simulink model "IEEE39bus"  (Simulink 8.5)
settings: Solver=ode3  SolverMode=SingleTasking  StartTime=0.0  StopTime=50  FixedStep=Ts  RelTol=1e-3
PostLoadFcn:
  | Ts=25e-6; IEEE39BusLineLength;
  | vNomHV = 345E3;fNom=50;load('Dynamicload.mat');
InitFcn:
  | Ts=25e-6; IEEE39BusLineLength;
  | vNomHV = 345E3;fNom=50;load('Dynamicload.mat');
undefined symbols (not defined in the file): D1, Delta, load15, load16, load18, load20, load21, load23, load24, load25, load26, load27, load28, load29, load3, load39, load4, load7, load8, TL_10_11_len, TL_10_13_len, TL_13_14_len, TL_14_15_len, TL_15_16_len, TL_16_17_len, TL_16_19_len, TL_16_21_len, TL_16_24_len, TL_17_18_len, TL_17_27_len, TL_1_2_len, TL_1_39_len, TL_21_22_len, TL_22_23_len, TL_24_23_len, TL_25_26_len, TL_26_27_len, TL_26_28_len, TL_26_29_len, TL_28_29_len, TL_2_25_len, TL_2_2_len, TL_3_18_len, TL_3_4_len, TL_4_14_len, TL_4_5_len, TL_5_6_len, TL_5_8_len, TL_6_11_len, TL_6_7_len, TL_7_8_len, TL_8_9_len, TL_9_39_len
libraries: powerlib x175, op_dpl_lib x34, rtlab x14, sps_avr x9, powerlib_extras x2, artemis x1, powerlib_meascontrol x1
(part 3 of 5)

== system IEEE39bus/SS_EastSystem1/GT 5 ==
  5 MW : powerlib/Elements/Three-Phase Parallel RLC Load  LConnTagsString=A|B|C  Configuration=Y (grounded)  NominalVoltage=22e3  NominalFrequency=50  ActivePower=5e6  InductivePower=0  CapacitivePower=0  Measurements=None  LoadType=constant Z
  Bus Selector1 : BusSelector  OutputSignals="dq0 components.Stator voltage  vq (pu),dq0 components.Stator voltage  vd (pu),Mechanical.Rotor speed  wm  (pu),Mechanical.Rotor speed deviation  dw (pu),Output active power   Peo (pu),Output reactive power  Qeo (pu)"
  Bus 34 : powerlib/Measurements/Three-Phase V-I Measurement  VoltageMeasurement=phase-to-ground  SetLabelV=on  LabelV=V_bus_G5  Vpu=off  VpuLL=off  CurrentMeasurement=no  SetLabelI=on  LabelI=I_bus_G5  Ipu=off  Pbase=100e6  Vbase=16.5e3  OutputType=Complex  PhasorSimulation=off  PSBequivalent=0
  Excitation System1 : sps_avr/Excitation System  tr=20e-3  reg=[ 200, 0.02 ]  exc=[ 1, 0 .19]  tgr=[ 0, 0 ]  damp=[ 0.0012, 1 ]  sat=[ 0, 0 ]  lim=[ 0, 7.32, 0 ]  v0=[1.0123 3.3412]
  GT1_CB6 : Subsystem
  Ground : Ground
  HTG : powerlib/Machines/Hydraulic Turbine and Governor  sm="[ 10/3  0.07 ]"  gate="[  0.01  0.97518  -0.1  0.1 ]"  reg="[  0.05  1.163  0.105  0  0.01  ]"  hyd="[  0  2.67  ]"  dref=0  po=0.709
  Load Flow Bus : powerlib/Measurements/Load Flow Bus  LConnTagsString=a  ID=Bus-34  Vbase=22000  Vref=1.0123  Vangle=0  VLF=1.012  angleLF=-37.01
      settings: AttributesFormatString=%<ID>\n%<Vbase>V\n%<VLF>pu\n%<angleLF>deg.
  Machine 5 520 MVA 22 kV : powerlib/Machines/Synchronous Machine pu Standard  PresetModel=No  MechanicalLoad=Mechanical power Pm  ShowDetailedParameters=on  RotorType=Round  Units=per unit standard parameters  MeasurementBus=off  NominalParameters="[ 520E6  22000   50 ]"  Reactances1=[ 3.484 0.686 0.343 3.224 0.8632 0.343 0.054 ]  Reactances2=[ 0.995, 0.195, 0.155, 0.568, 0.143, 0.16 ]  dAxisTimeConstants=Open-circuit  qAxisTimeConstants=Open-circuit  TimeConstants1=[]  TimeConstants2=[5.4 0.03 0.44 0.04]  TimeConstants3=[]  TimeConstants4=[]  TimeConstants5=[ 9.2, 0.01, 0.01 ]  TimeConstants6=[]  TimeConstants7=[]  TimeConstants8=[]  StatorResistance=0  Mechanical=[ 5 0.02 20]  PolePairs=20  InitialConditions=[0 -74.2196 0.822255 0.822255 0.822255 -56.5136 -176.514 63.4864 3.34118]  SetSaturation=off  Saturation=[0.6404,0.7127,0.8441,0.9214,0.9956,1.082,1.19,1.316,1.457;0.7,0.7698,0.8872,0.9466,0.9969,1.046,1.1,1.151,1.201]  LoadFlowParameters=[1 508000000 22270.6 0]  TsPowergui=0  TsBlock=-1  IterativeModel=Trapezoidal non iterative  BusType=PV  Pref=4.08e+008  Qref=0  Qmin=-300e6  Qmax=200e6  PLF=0  QLF=0
      settings: AttributesFormatString=\n\n
  Pref : Constant  Value=0.709
  Terminator5 : Terminator
  Transformer 5 572 MVA 22 kV / 345 kV : powerlib/Elements/Three-Phase Transformer (Two Windings)  Winding1Connection=Delta (D1)  Winding2Connection=Yg  CoreType=Three single-phase transformers  SetSaturation=off  Hysteresis=off  DataFile='hysteresis'  SetInitialFlux=off  Measurements=None  UNITS=pu  NominalPower=[ 572e6 50 ]  Winding1="[ 22e3 0.009*572/100/2    0.018*572/100/2]"  Winding2="[ 1.009*345e3 0.009*572/100/2    0.018*572/100/2]"  Rm=500  Lm=500  L0=0.5  Saturation="[ 0,0  ;  0.005,1.2  ;  1.0,1.4 ]"  InitialFluxes=[ 0.8 , -0.8 , 0.7 ]  MoreParameters=off  BreakLoop=off  DataType=off  TransfoNumber=0
  Vref : Constant  Value=1.0123
  wref : Constant
  A : PMIOPort  Port=1  Side=Right
  B : PMIOPort  Port=2  Side=Right
  C : PMIOPort  Port=3  Side=Right
  tag scope: P_G5=global, Q_G5=global, V_G5=global, Wm_G5=global
  wires:
  Ground/1 -> Excitation System1/4
  HTG/2 -> Terminator5/1
  Vref/1 -> Excitation System1/1
  Pref/1 -> HTG/2
  wref/1 -> HTG/1
  HTG/1 -> Machine 5 520 MVA 22 kV/1
  Machine 5 520 MVA 22 kV/1 -> Bus Selector1/1
  Bus Selector1/1 -> Excitation System1/3  "<Stator voltage  vq (pu)>"
  Bus Selector1/2 -> Excitation System1/2  "<Stator voltage  vd (pu)>"
  Bus Selector1/3 -> HTG/3, [Wm_G5]  "<Rotor speed  wm  (pu)>"
  Bus Selector1/4 -> HTG/5  "<Rotor speed deviation  dw (pu)>"
  Bus Selector1/5 -> HTG/4, [P_G5]  "<Output active power   Peo (pu)>"
  Bus Selector1/6 -> [Q_G5]  "<Output reactive power  Qeo (pu)>"
  [V_bus_G5] -> [V_G5]
  Excitation System1/1 -> Machine 5 520 MVA 22 kV/2
  connections:
  Transformer 5 572 MVA 22 kV / 345 kV/LConn1 -- Load Flow Bus/LConn1 -- Bus 34/RConn1 -- 5 MW/LConn1
  Transformer 5 572 MVA 22 kV / 345 kV/LConn2 -- Bus 34/RConn2 -- 5 MW/LConn2
  Transformer 5 572 MVA 22 kV / 345 kV/LConn3 -- Bus 34/RConn3 -- 5 MW/LConn3
  Machine 5 520 MVA 22 kV/RConn1 -- Bus 34/LConn1
  Machine 5 520 MVA 22 kV/RConn2 -- Bus 34/LConn2
  Machine 5 520 MVA 22 kV/RConn3 -- Bus 34/LConn3
  GT1_CB6/LConn1 -- Transformer 5 572 MVA 22 kV / 345 kV/RConn1
  GT1_CB6/LConn2 -- Transformer 5 572 MVA 22 kV / 345 kV/RConn2
  GT1_CB6/LConn3 -- Transformer 5 572 MVA 22 kV / 345 kV/RConn3
  B/RConn1 -- GT1_CB6/RConn2
  A/RConn1 -- GT1_CB6/RConn1
  C/RConn1 -- GT1_CB6/RConn3

== system IEEE39bus/SS_EastSystem1/Load 15 ==
  Bus_L15 : powerlib/Measurements/Three-Phase V-I Measurement  VoltageMeasurement=phase-to-ground  SetLabelV=off  LabelV=V_Bus_L15  Vpu=off  VpuLL=off  CurrentMeasurement=yes  SetLabelI=on  LabelI=I_L15  Ipu=off  Pbase=100e6  Vbase=230e3  OutputType=Complex  PhasorSimulation=off  PSBequivalent=0
  Terminator : Terminator
  Three-Phase Dynamic Load : powerlib/Elements/Three-Phase Dynamic Load  NominalVoltage=[345e3 50 ]  ActiveReactivePowers=[3.2e+08 1.53e+08]  PositiveSequence=[0.99604 18.5295]  ExternalControl=on  NpNq=[0 0]  TimeConstants="[0  0  0  0]"  MinimumVoltage=0.7  LoadFlowParameters=[4,0,0,0,0]
  A : PMIOPort  Port=1  Side=Left
  B : PMIOPort  Port=2  Side=Left
  C : PMIOPort  Port=3  Side=Left
  tag scope: V_L15=global
  wires:
  Three-Phase Dynamic Load/1 -> Terminator/1
  Bus_L15/1 -> [V_L15]
  [load15] -> Three-Phase Dynamic Load/1
  connections:
  C/RConn1 -- Bus_L15/LConn3
  Bus_L15/RConn3 -- Three-Phase Dynamic Load/LConn3
  Bus_L15/RConn2 -- Three-Phase Dynamic Load/LConn2
  A/RConn1 -- Bus_L15/LConn1
  B/RConn1 -- Bus_L15/LConn2
  Bus_L15/RConn1 -- Three-Phase Dynamic Load/LConn1

== system IEEE39bus/SS_EastSystem1/Load 16 ==
  Bus_L16 : powerlib/Measurements/Three-Phase V-I Measurement  VoltageMeasurement=phase-to-ground  SetLabelV=off  LabelV=V_Bus_L16  Vpu=off  VpuLL=off  CurrentMeasurement=yes  SetLabelI=on  LabelI=I_L16  Ipu=off  Pbase=100e6  Vbase=230e3  OutputType=Complex  PhasorSimulation=off  PSBequivalent=0
  Terminator : Terminator
  Three-Phase Dynamic Load : powerlib/Elements/Three-Phase Dynamic Load  NominalVoltage=[345e3 50 ]  ActiveReactivePowers=[3.29e+08 3.23e+07]  PositiveSequence=[1.00736 19.2229]  ExternalControl=on  NpNq=[0 0]  TimeConstants="[0  0  0  0]"  MinimumVoltage=0.7  LoadFlowParameters=[4,0,0,0,0]
  A : PMIOPort  Port=1  Side=Left
  B : PMIOPort  Port=2  Side=Left
  C : PMIOPort  Port=3  Side=Left
  tag scope: V_L16=global
  wires:
  Three-Phase Dynamic Load/1 -> Terminator/1
  Bus_L16/1 -> [V_L16]
  [load16] -> Three-Phase Dynamic Load/1
  connections:
  Three-Phase Dynamic Load/LConn1 -- Bus_L16/RConn1
  C/RConn1 -- Bus_L16/LConn3
  B/RConn1 -- Bus_L16/LConn2
  A/RConn1 -- Bus_L16/LConn1
  Bus_L16/RConn2 -- Three-Phase Dynamic Load/LConn2
  Bus_L16/RConn3 -- Three-Phase Dynamic Load/LConn3

== system IEEE39bus/SS_EastSystem1/Load 20 ==
  Bus_L20 : powerlib/Measurements/Three-Phase V-I Measurement  VoltageMeasurement=phase-to-ground  SetLabelV=off  LabelV=V_Bus_L20  Vpu=off  VpuLL=off  CurrentMeasurement=yes  SetLabelI=on  LabelI=I_L20  Ipu=off  Pbase=100e6  Vbase=230e3  OutputType=Complex  PhasorSimulation=off  PSBequivalent=0
  Snubber : powerlib/Elements/Three-Phase Series RLC Load  LConnTagsString=A|B|C  Configuration=Y (grounded)  NominalVoltage=345E3  NominalFrequency=50  ActivePower=1e6  InductivePower=0  CapacitivePower=1e7  Measurements=None  LoadType=constant Z
  Terminator : Terminator
  Three-Phase Dynamic Load : powerlib/Elements/Three-Phase Dynamic Load  NominalVoltage=[345e3 50 ]  ActiveReactivePowers=[6.28e+08 1.03e+08]  PositiveSequence=[0.961329 -10.5466]  ExternalControl=on  NpNq=[0 0]  TimeConstants="[0  0  0  0]"  MinimumVoltage=0.7  LoadFlowParameters=[4,0,0,0,0]
  A : PMIOPort  Port=1  Side=Left
  B : PMIOPort  Port=2  Side=Left
  C : PMIOPort  Port=3  Side=Left
  tag scope: V_L20=global
  wires:
  Three-Phase Dynamic Load/1 -> Terminator/1
  Bus_L20/1 -> [V_L20]
  [load20] -> Three-Phase Dynamic Load/1
  connections:
  Bus_L20/RConn3 -- Snubber/LConn3 -- Three-Phase Dynamic Load/LConn3
  Bus_L20/RConn2 -- Snubber/LConn2 -- Three-Phase Dynamic Load/LConn2
  A/RConn1 -- Bus_L20/LConn1
  B/RConn1 -- Bus_L20/LConn2
  C/RConn1 -- Bus_L20/LConn3
  Bus_L20/RConn1 -- Snubber/LConn1 -- Three-Phase Dynamic Load/LConn1

== system IEEE39bus/SS_EastSystem1/Machines Measurements ==
  Mux : Mux  Inputs=2
  Mux1 : Mux
  Mux2 : Mux
  Machines Measurements : Outport
  wires:
  Mux2/1 -> Mux/2
  Mux1/1 -> Mux/1
  Mux/1 -> Machines Measurements/1
  [Wm_G5] -> Mux2/4
  [Q_G5] -> Mux2/3
  [P_G5] -> Mux2/2
  [V_G5] -> Mux2/1
  [Wm_G4] -> Mux1/4
  [Q_G4] -> Mux1/3
  [P_G4] -> Mux1/2
  [V_G4] -> Mux1/1

== system IEEE39bus/SS_EastSystem2/Buses current_E ==
  Mux3 : Mux
  current : Outport
  wires:
  Mux3/1 -> current/1
  [I_L21] -> Mux3/1
  [I_bus_22] -> Mux3/2
  [I_L23] -> Mux3/3
  [I_L24] -> Mux3/4

== system IEEE39bus/SS_EastSystem2/Buses voltages_E ==
  Mux3 : Mux
  Voltages : Outport
  wires:
  [V_L24] -> Mux3/4
  [V_L23] -> Mux3/3
  [V_bus_22] -> Mux3/2
  [V_L21] -> Mux3/1
  Mux3/1 -> Voltages/1

== system IEEE39bus/SS_EastSystem2/GT 6 ==
  5 MW : powerlib/Elements/Three-Phase Parallel RLC Load  LConnTagsString=A|B|C  Configuration=Y (grounded)  NominalVoltage=22e3  NominalFrequency=50  ActivePower=5e6  InductivePower=0  CapacitivePower=0  Measurements=None  LoadType=constant Z
  Bus Selector1 : BusSelector  OutputSignals="dq0 components.Stator voltage  vq (pu),dq0 components.Stator voltage  vd (pu),Mechanical.Rotor speed  wm  (pu),Mechanical.Rotor speed deviation  dw (pu),Output active power   Peo (pu),Output reactive power  Qeo (pu)"
  Bus 35 : powerlib/Measurements/Three-Phase V-I Measurement  VoltageMeasurement=phase-to-ground  SetLabelV=on  LabelV=V_bus_G6  Vpu=off  VpuLL=off  CurrentMeasurement=no  SetLabelI=on  LabelI=I_bus_G6  Ipu=off  Pbase=100e6  Vbase=16.5e3  OutputType=Complex  PhasorSimulation=off  PSBequivalent=0
  Excitation System : sps_avr/Excitation System  tr=20e-3  reg=[ 200, 0.02 ]  exc=[ 1, 0 .19]  tgr=[ 0, 0 ]  damp=[ 0.0012, 1 ]  sat=[ 0, 0 ]  lim=[ 0, 7.32, 0 ]  v0=[1.02 1.8033]
  GT1_CB8 : Subsystem
  Ground : Ground
  HTG : powerlib/Machines/Hydraulic Turbine and Governor  sm="[ 10/3  0.07 ]"  gate="[  0.01  0.97518  -0.1  0.1 ]"  reg="[  0.05  1.163  0.105  0  0.01  ]"  hyd="[  0  2.67  ]"  dref=0  po=0.51
  Load Flow Bus : powerlib/Measurements/Load Flow Bus  LConnTagsString=a  ID=Bus-35  Vbase=22000  Vref=1.02  Vangle=0  VLF=1.02  angleLF=-1.943
      settings: AttributesFormatString=%<ID>\n%<Vbase>V\n%<VLF>pu\n%<angleLF>deg.
  Machine 6 1000 MVA 22 kV : powerlib/Machines/Synchronous Machine pu Standard  PresetModel=No  MechanicalLoad=Mechanical power Pm  ShowDetailedParameters=on  RotorType=Round  Units=per unit standard parameters  MeasurementBus=off  NominalParameters="[ 1000E6  22000   50 ]"  Reactances1=[ 2.032 0.4 0.2 1.928 0.651 0.2 0.022 ]  Reactances2=[ 0.995, 0.195, 0.155, 0.568, 0.143, 0.16 ]  dAxisTimeConstants=Open-circuit  qAxisTimeConstants=Open-circuit  TimeConstants1=[]  TimeConstants2=[7.3 0.03 0.4 0.04]  TimeConstants3=[]  TimeConstants4=[]  TimeConstants5=[ 9.2, 0.01, 0.01 ]  TimeConstants6=[]  TimeConstants7=[]  TimeConstants8=[]  StatorResistance=0.005  Mechanical=[ 4.35 0.02 20]  PolePairs=20  InitialConditions=[0 -55.6147 0.575854 0.575854 0.575854 -22.492 -142.492 97.508 1.80331]  SetSaturation=off  Saturation=[0.6404,0.7127,0.8441,0.9214,0.9956,1.082,1.19,1.316,1.457;0.7,0.7698,0.8872,0.9466,0.9969,1.046,1.1,1.151,1.201]  LoadFlowParameters=[1 650000000 23084.6 0]  TsPowergui=0  TsBlock=-1  IterativeModel=Trapezoidal non iterative  BusType=PV  Pref=5.50e+008  Qref=0  Qmin=-500e6  Qmax=250e6  PLF=0  QLF=0
      settings: AttributesFormatString=\n\n
  Pref : Constant  Value=0.51
  Terminator5 : Terminator
  Transformer 6 880 MVA 22  kV / 345 kV : powerlib/Elements/Three-Phase Transformer (Two Windings)  Winding1Connection=Delta (D1)  Winding2Connection=Yg  CoreType=Three single-phase transformers  SetSaturation=off  Hysteresis=off  DataFile='hysteresis'  SetInitialFlux=off  Measurements=None  UNITS=pu  NominalPower=[ 880e6 50 ]  Winding1="[ 22e3  0.0   0.0143*880/100/2]"  Winding2="[ 1.025*345e3 0.0   0.0143*880/100/2]"  Rm=500  Lm=500  L0=0.5  Saturation="[ 0,0  ;  0.005,1.2  ;  1.0,1.4 ]"  InitialFluxes=[ 0.8 , -0.8 , 0.7 ]  MoreParameters=off  BreakLoop=off  DataType=off  TransfoNumber=0
  Vref : Constant  Value=1.02
  wref : Constant
  A : PMIOPort  Port=1  Side=Right
  B : PMIOPort  Port=2  Side=Right
  C : PMIOPort  Port=3  Side=Right
  tag scope: P_G6=global, Q_G6=global, V_G6=global, Wm_G6=global
  wires:
  Ground/1 -> Excitation System/4
  HTG/2 -> Terminator5/1
  Vref/1 -> Excitation System/1
  Pref/1 -> HTG/2
  wref/1 -> HTG/1
  Excitation System/1 -> Machine 6 1000 MVA 22 kV/2
  HTG/1 -> Machine 6 1000 MVA 22 kV/1
  Machine 6 1000 MVA 22 kV/1 -> Bus Selector1/1
  Bus Selector1/1 -> Excitation System/3  "<Stator voltage  vq (pu)>"
  Bus Selector1/2 -> Excitation System/2  "<Stator voltage  vd (pu)>"
  Bus Selector1/3 -> HTG/3, [Wm_G6]  "<Rotor speed  wm  (pu)>"
  Bus Selector1/4 -> HTG/5  "<Rotor speed deviation  dw (pu)>"
  Bus Selector1/5 -> HTG/4, [P_G6]  "<Output active power   Peo (pu)>"
  Bus Selector1/6 -> [Q_G6]  "<Output reactive power  Qeo (pu)>"
  [V_bus_G6] -> [V_G6]
  connections:
  Transformer 6 880 MVA 22  kV / 345 kV/LConn1 -- Load Flow Bus/LConn1 -- Bus 35/RConn1 -- 5 MW/LConn1
  Transformer 6 880 MVA 22  kV / 345 kV/LConn2 -- Bus 35/RConn2 -- 5 MW/LConn2
  Transformer 6 880 MVA 22  kV / 345 kV/LConn3 -- Bus 35/RConn3 -- 5 MW/LConn3
  Machine 6 1000 MVA 22 kV/RConn1 -- Bus 35/LConn1
  Machine 6 1000 MVA 22 kV/RConn2 -- Bus 35/LConn2
  Machine 6 1000 MVA 22 kV/RConn3 -- Bus 35/LConn3
  GT1_CB8/LConn1 -- Transformer 6 880 MVA 22  kV / 345 kV/RConn1
  GT1_CB8/LConn2 -- Transformer 6 880 MVA 22  kV / 345 kV/RConn2
  GT1_CB8/LConn3 -- Transformer 6 880 MVA 22  kV / 345 kV/RConn3
  B/RConn1 -- GT1_CB8/RConn2
  A/RConn1 -- GT1_CB8/RConn1
  C/RConn1 -- GT1_CB8/RConn3

== system IEEE39bus/SS_EastSystem2/GT 7 ==
  5 MW : powerlib/Elements/Three-Phase Parallel RLC Load  LConnTagsString=A|B|C  Configuration=Y (grounded)  NominalVoltage=22e3  NominalFrequency=50  ActivePower=5e6  InductivePower=0  CapacitivePower=0  Measurements=None  LoadType=constant Z
  Bus Selector1 : BusSelector  OutputSignals="dq0 components.Stator voltage  vq (pu),dq0 components.Stator voltage  vd (pu),Mechanical.Rotor speed  wm  (pu),Mechanical.Rotor speed deviation  dw (pu),Output active power   Peo (pu),Output reactive power  Qeo (pu)"
  Bus 36 : powerlib/Measurements/Three-Phase V-I Measurement  VoltageMeasurement=phase-to-ground  SetLabelV=on  LabelV=V_bus_G7  Vpu=off  VpuLL=off  CurrentMeasurement=no  SetLabelI=on  LabelI=I_bus_G7  Ipu=off  Pbase=100e6  Vbase=16.5e3  OutputType=Complex  PhasorSimulation=off  PSBequivalent=0
  Excitation System : sps_avr/Excitation System  tr=20e-3  reg=[ 200, 0.02 ]  exc=[ 1, 0 .19]  tgr=[ 0, 0 ]  damp=[ 0.0012, 1 ]  sat=[ 0, 0 ]  lim=[ 0, 7.32, 0 ]  v0=[1.015 1.5412]
  GT1_CB10 : Subsystem
  Ground : Ground
  HTG : powerlib/Machines/Hydraulic Turbine and Governor  sm="[ 10/3  0.07 ]"  gate="[  0.01  0.97518  -0.1  0.1 ]"  reg="[  0.05  1.163  0.105  0  0.01  ]"  hyd="[  0  2.67  ]"  dref=0  po=0.42
  Load Flow Bus : powerlib/Measurements/Load Flow Bus  LConnTagsString=a  ID=Bus-36  Vbase=22000  Vref=1.015  Vangle=0  VLF=1.015  angleLF=0.3154
      settings: AttributesFormatString=%<ID>\n%<Vbase>V\n%<VLF>pu\n%<angleLF>deg.
  Machine 7 1000 MVA 22 kV : powerlib/Machines/Synchronous Machine pu Standard  PresetModel=No  MechanicalLoad=Mechanical power Pm  ShowDetailedParameters=on  RotorType=Round  Units=per unit standard parameters  MeasurementBus=off  NominalParameters="[ 1000E6  22000   50 ]"  Reactances1=[ 2.408 0.4 0.2 2.384 1.518 0.2 0.032 ]  Reactances2=[ 0.995, 0.195, 0.155, 0.568, 0.143, 0.16 ]  dAxisTimeConstants=Open-circuit  qAxisTimeConstants=Open-circuit  TimeConstants1=[]  TimeConstants2=[5.66 0.03 1.5 0.04]  TimeConstants3=[]  TimeConstants4=[]  TimeConstants5=[ 9.2, 0.01, 0.01 ]  TimeConstants6=[]  TimeConstants7=[]  TimeConstants8=[]  StatorResistance=0.005  Mechanical=[ 3.23 0.02 20]  PolePairs=20  InitialConditions=[0 -44.8827 0.454166 0.454166 0.454166 -3.41889 -123.419 116.581 1.54123]  SetSaturation=off  Saturation=[0.6404,0.7127,0.8441,0.9214,0.9956,1.082,1.19,1.316,1.457;0.7,0.7698,0.8872,0.9466,0.9969,1.046,1.1,1.151,1.201]  LoadFlowParameters=[1 560000000 23397 0]  TsPowergui=0  TsBlock=-1  IterativeModel=Trapezoidal non iterative  BusType=PV  Pref=4.6e+008  Qref=0  Qmin=-500e6  Qmax=150e6  PLF=0  QLF=0
      settings: AttributesFormatString=\n\n
  Pref : Constant  Value=0.42
  Terminator5 : Terminator
  Transformer 7 897.6 MVA 22 kV / 345 kV : powerlib/Elements/Three-Phase Transformer (Two Windings)  Winding1Connection=Delta (D1)  Winding2Connection=Yg  CoreType=Three single-phase transformers  SetSaturation=off  Hysteresis=off  DataFile='hysteresis'  SetInitialFlux=off  Measurements=None  UNITS=pu  NominalPower=[ 897.6e6 50]  Winding1="[ 22e3  0.0005*897.6/100/2     0.0272*897.6/100/2]"  Winding2="[ 345e3 0.0005*897.6/100/2     0.0272*897.6/100/2]"  Rm=500  Lm=500  L0=0.5  Saturation="[ 0,0  ;  0.005,1.2  ;  1.0,1.4 ]"  InitialFluxes=[ 0.8 , -0.8 , 0.7 ]  MoreParameters=off  BreakLoop=off  DataType=off  TransfoNumber=0
  Vref : Constant  Value=1.015
  wref : Constant
  A : PMIOPort  Port=1  Side=Right
  B : PMIOPort  Port=2  Side=Right
  C : PMIOPort  Port=3  Side=Right
  tag scope: P_G7=global, Q_G7=global, V_G7=global, Wm_G7=global
  wires:
  Ground/1 -> Excitation System/4
  HTG/2 -> Terminator5/1
  Vref/1 -> Excitation System/1
  Pref/1 -> HTG/2
  wref/1 -> HTG/1
  Excitation System/1 -> Machine 7 1000 MVA 22 kV/2
  HTG/1 -> Machine 7 1000 MVA 22 kV/1
  Machine 7 1000 MVA 22 kV/1 -> Bus Selector1/1
  Bus Selector1/1 -> Excitation System/3  "<Stator voltage  vq (pu)>"
  Bus Selector1/2 -> Excitation System/2  "<Stator voltage  vd (pu)>"
  Bus Selector1/3 -> HTG/3, [Wm_G7]  "<Rotor speed  wm  (pu)>"
  Bus Selector1/4 -> HTG/5  "<Rotor speed deviation  dw (pu)>"
  Bus Selector1/5 -> HTG/4, [P_G7]  "<Output active power   Peo (pu)>"
  Bus Selector1/6 -> [Q_G7]  "<Output reactive power  Qeo (pu)>"
  [V_bus_G7] -> [V_G7]
  connections:
  Transformer 7 897.6 MVA 22 kV / 345 kV/LConn1 -- Load Flow Bus/LConn1 -- Bus 36/RConn1 -- 5 MW/LConn1
  Transformer 7 897.6 MVA 22 kV / 345 kV/LConn2 -- Bus 36/RConn2 -- 5 MW/LConn2
  Transformer 7 897.6 MVA 22 kV / 345 kV/LConn3 -- Bus 36/RConn3 -- 5 MW/LConn3
  Machine 7 1000 MVA 22 kV/RConn1 -- Bus 36/LConn1
  Machine 7 1000 MVA 22 kV/RConn2 -- Bus 36/LConn2
  Machine 7 1000 MVA 22 kV/RConn3 -- Bus 36/LConn3
  GT1_CB10/LConn3 -- Transformer 7 897.6 MVA 22 kV / 345 kV/RConn3
  GT1_CB10/LConn2 -- Transformer 7 897.6 MVA 22 kV / 345 kV/RConn2
  GT1_CB10/LConn1 -- Transformer 7 897.6 MVA 22 kV / 345 kV/RConn1
  B/RConn1 -- GT1_CB10/RConn2
  A/RConn1 -- GT1_CB10/RConn1
  C/RConn1 -- GT1_CB10/RConn3

== system IEEE39bus/SS_EastSystem2/Load 21 ==
  Bus_L21 : powerlib/Measurements/Three-Phase V-I Measurement  VoltageMeasurement=phase-to-ground  SetLabelV=off  LabelV=V_Bus_L21  Vpu=off  VpuLL=off  CurrentMeasurement=yes  SetLabelI=on  LabelI=I_L21  Ipu=off  Pbase=100e6  Vbase=230e3  OutputType=Complex  PhasorSimulation=off  PSBequivalent=0
  Terminator : Terminator
  Three-Phase Dynamic Load : powerlib/Elements/Three-Phase Dynamic Load  NominalVoltage=[345e3 50 ]  ActiveReactivePowers=[2.74e+08 1.15e+08]  PositiveSequence=[1.00586 20.5637]  ExternalControl=on  NpNq=[0 0]  TimeConstants="[0  0  0  0]"  MinimumVoltage=0.7  LoadFlowParameters=[4,0,0,0,0]
  A : PMIOPort  Port=1  Side=Left
  B : PMIOPort  Port=2  Side=Left
  C : PMIOPort  Port=3  Side=Left
  tag scope: V_L21=global
  wires:
  Three-Phase Dynamic Load/1 -> Terminator/1
  Bus_L21/1 -> [V_L21]
  [load21] -> Three-Phase Dynamic Load/1
  connections:
  Bus_L21/RConn1 -- Three-Phase Dynamic Load/LConn1
  C/RConn1 -- Bus_L21/LConn3
  B/RConn1 -- Bus_L21/LConn2
  A/RConn1 -- Bus_L21/LConn1
  Bus_L21/RConn2 -- Three-Phase Dynamic Load/LConn2
  Bus_L21/RConn3 -- Three-Phase Dynamic Load/LConn3

== system IEEE39bus/SS_EastSystem2/Load 23 ==
  Bus_L23 : powerlib/Measurements/Three-Phase V-I Measurement  VoltageMeasurement=phase-to-ground  SetLabelV=off  LabelV=V_Bus_L23  Vpu=off  VpuLL=off  CurrentMeasurement=yes  SetLabelI=on  LabelI=I_L23  Ipu=off  Pbase=100e6  Vbase=230e3  OutputType=Complex  PhasorSimulation=off  PSBequivalent=0
  Terminator : Terminator
  Three-Phase Dynamic Load : powerlib/Elements/Three-Phase Dynamic Load  NominalVoltage=[345e3 50]  ActiveReactivePowers=[2.475e+08 8.46e+07]  PositiveSequence=[1.0123 23.421]  ExternalControl=on  NpNq=[0 0]  TimeConstants="[0  0  0  0]"  MinimumVoltage=0.7  LoadFlowParameters=[4,0,0,0,0]
  A : PMIOPort  Port=1  Side=Left
  B : PMIOPort  Port=2  Side=Left
  C : PMIOPort  Port=3  Side=Left
  tag scope: V_L23=global
  wires:
  Three-Phase Dynamic Load/1 -> Terminator/1
  Bus_L23/1 -> [V_L23]
  [load23] -> Three-Phase Dynamic Load/1
  connections:
  Three-Phase Dynamic Load/LConn1 -- Bus_L23/RConn1
  C/RConn1 -- Bus_L23/LConn3
  B/RConn1 -- Bus_L23/LConn2
  A/RConn1 -- Bus_L23/LConn1
  Three-Phase Dynamic Load/LConn2 -- Bus_L23/RConn2
  Three-Phase Dynamic Load/LConn3 -- Bus_L23/RConn3

== system IEEE39bus/SS_EastSystem2/Load 24 ==
  Bus_L24 : powerlib/Measurements/Three-Phase V-I Measurement  VoltageMeasurement=phase-to-ground  SetLabelV=off  LabelV=V_Bus_L24  Vpu=off  VpuLL=off  CurrentMeasurement=yes  SetLabelI=on  LabelI=I_L24  Ipu=off  Pbase=100e6  Vbase=230e3  OutputType=Complex  PhasorSimulation=off  PSBequivalent=0
  Terminator : Terminator
  Three-Phase Dynamic Load : powerlib/Elements/Three-Phase Dynamic Load  NominalVoltage=[345e3 50 ]  ActiveReactivePowers=[3.086e+08 -9.2e+07]  PositiveSequence=[1.01137 19.0799]  ExternalControl=on  NpNq=[0 0]  TimeConstants="[0  0  0  0]"  MinimumVoltage=0.7  LoadFlowParameters=[4,0,0,0,0]
  A : PMIOPort  Port=1  Side=Left
  B : PMIOPort  Port=2  Side=Left
  C : PMIOPort  Port=3  Side=Left
  tag scope: V_L24=global
  wires:
  Three-Phase Dynamic Load/1 -> Terminator/1
  Bus_L24/1 -> [V_L24]
  [load24] -> Three-Phase Dynamic Load/1
  connections:
  Three-Phase Dynamic Load/LConn3 -- Bus_L24/RConn3
  Three-Phase Dynamic Load/LConn2 -- Bus_L24/RConn2
  A/RConn1 -- Bus_L24/LConn1
  B/RConn1 -- Bus_L24/LConn2
  C/RConn1 -- Bus_L24/LConn3
  Three-Phase Dynamic Load/LConn1 -- Bus_L24/RConn1

== system IEEE39bus/SS_EastSystem2/Machines Measurements ==
  Mux : Mux  Inputs=2
  Mux3 : Mux
  Mux4 : Mux
  Machines Measurements : Outport
  wires:
  Mux4/1 -> Mux/2
  Mux3/1 -> Mux/1
  [Wm_G7] -> Mux4/4
  [Q_G7] -> Mux4/3
  [P_G7] -> Mux4/2
  [V_G7] -> Mux4/1
  [Wm_G6] -> Mux3/4
  [Q_G6] -> Mux3/3
  [P_G6] -> Mux3/2
  [V_G6] -> Mux3/1
  Mux/1 -> Machines Measurements/1

== system IEEE39bus/SS_NorthSystem1/Buses current_N ==
  Mux3 : Mux
  curremt : Outport
  wires:
  [I_L25] -> Mux3/1
  [I_L26] -> Mux3/2
  [I_L28] -> Mux3/3
  [I_L29] -> Mux3/4
  Mux3/1 -> curremt/1

== system IEEE39bus/SS_NorthSystem1/Buses voltages_N ==
  Mux3 : Mux
  Voltages : Outport
  wires:
  Mux3/1 -> Voltages/1
  [V_L25] -> Mux3/1
  [V_L26] -> Mux3/2
  [V_L28] -> Mux3/3
  [V_L29] -> Mux3/4

== system IEEE39bus/SS_NorthSystem1/GT 8 ==
  5 MW : powerlib/Elements/Three-Phase Parallel RLC Load  LConnTagsString=A|B|C  Configuration=Y (grounded)  NominalVoltage=22e3  NominalFrequency=50  ActivePower=5e6  InductivePower=0  CapacitivePower=0  Measurements=None  LoadType=constant Z
  Bus Selector1 : BusSelector  OutputSignals="dq0 components.Stator voltage  vq (pu),dq0 components.Stator voltage  vd (pu),Mechanical.Rotor speed  wm  (pu),Mechanical.Rotor speed deviation  dw (pu),Output active power   Peo (pu),Output reactive power  Qeo (pu)"
  Bus 37 : powerlib/Measurements/Three-Phase V-I Measurement  VoltageMeasurement=phase-to-ground  SetLabelV=on  LabelV=V_bus_G8  Vpu=off  VpuLL=off  CurrentMeasurement=no  SetLabelI=on  LabelI=I_bus_G8  Ipu=off  Pbase=100e6  Vbase=16.5e3  OutputType=Complex  PhasorSimulation=off  PSBequivalent=0
  Excitation System : sps_avr/Excitation System  tr=20e-3  reg=[ 200, 0.02 ]  exc=[ 1, 0 .19]  tgr=[ 0, 0 ]  damp=[ 0.0012, 1 ]  sat=[ 0, 0 ]  lim=[ 0, 7.32, 0 ]  v0=[1.01 1.6849]
  GT1_CB11 : Subsystem
  Ground : Ground
  HTG : powerlib/Machines/Hydraulic Turbine and Governor  sm="[ 10/3  0.07 ]"  gate="[  0.01  0.97518  -0.1  0.1 ]"  reg="[  0.05  1.163  0.105  0  0.01  ]"  hyd="[  0  2.67  ]"  dref=0  po=0.6
  Load Flow Bus : powerlib/Measurements/Load Flow Bus  LConnTagsString=a  ID=Bus-37  Vbase=22000  Vref=1.01  Vangle=0  VLF=1.01  angleLF=3.342
      settings: AttributesFormatString=%<ID>\n%<Vbase>V\n%<VLF>pu\n%<angleLF>deg.
  Machine 8 1000 MVA 22 kV : powerlib/Machines/Synchronous Machine pu Standard  PresetModel=No  MechanicalLoad=Mechanical power Pm  ShowDetailedParameters=on  RotorType=Round  Units=per unit standard parameters  MeasurementBus=off  NominalParameters="[ 1000E6  22000   50 ]"  Reactances1=[ 2.035 0.4 0.2 1.965 0.639 0.2 0.028 ]  Reactances2=[ 0.995, 0.195, 0.155, 0.568, 0.143, 0.16 ]  dAxisTimeConstants=Open-circuit  qAxisTimeConstants=Open-circuit  TimeConstants1=[]  TimeConstants2=[6.7 0.03 0.41 0.04]  TimeConstants3=[]  TimeConstants4=[]  TimeConstants5=[ 9.2, 0.01, 0.01 ]  TimeConstants6=[]  TimeConstants7=[]  TimeConstants8=[]  StatorResistance=0.005  Mechanical=[ 3.46 0.02 20]  PolePairs=20  InitialConditions=[0 -37.6671 0.634647 0.634647 0.634647 0.151083 -119.849 120.151 1.68493]  SetSaturation=off  Saturation=[0.6404,0.7127,0.8441,0.9214,0.9956,1.082,1.19,1.316,1.457;0.7,0.7698,0.8872,0.9466,0.9969,1.046,1.1,1.151,1.201]  LoadFlowParameters=[1 540000000 22611.6 0]  TsPowergui=0  TsBlock=-1  IterativeModel=Trapezoidal non iterative  BusType=PV  Pref=6.4e+008  Qref=0  Qmin=-500e6  Qmax=50e6  PLF=0  QLF=0
      settings: AttributesFormatString=\n\n
  Pref : Constant  Value=0.6
  Terminator5 : Terminator
  Transformer 8 772.2 MVA 22 kV / 345 kV : powerlib/Elements/Three-Phase Transformer (Two Windings)  Winding1Connection=Delta (D1)  Winding2Connection=Yg  CoreType=Three single-phase transformers  SetSaturation=off  Hysteresis=off  DataFile='hysteresis'  SetInitialFlux=off  Measurements=None  UNITS=pu  NominalPower=[ 1000e6 50 ]  Winding1="[ 22e3    0.0006*1000/100/2  0.0232*1000/100/2 ]"  Winding2="[ 1.025*345e3    0.0006*1000/100/2  0.0232*1000/100/2  ]"  Rm=500  Lm=500  L0=0.5  Saturation="[ 0,0  ;  0.005,1.2  ;  1.0,1.4 ]"  InitialFluxes=[ 0.8 , -0.8 , 0.7 ]  MoreParameters=off  BreakLoop=off  DataType=off  TransfoNumber=0
  Vref : Constant  Value=1.01
  wref : Constant
  A : PMIOPort  Port=1  Side=Right
  B : PMIOPort  Port=2  Side=Right
  C : PMIOPort  Port=3  Side=Right
  tag scope: P_G8=global, Q_G8=global, V_G8=global, Wm_G8=global
  wires:
  [V_bus_G8] -> [V_G8]
  Bus Selector1/6 -> [Q_G8]  "<Output reactive power  Qeo (pu)>"
  Bus Selector1/5 -> [P_G8], HTG/4  "<Output active power   Peo (pu)>"
  Bus Selector1/4 -> HTG/5  "<Rotor speed deviation  dw (pu)>"
  Bus Selector1/3 -> [Wm_G8], HTG/3  "<Rotor speed  wm  (pu)>"
  Bus Selector1/2 -> Excitation System/2  "<Stator voltage  vd (pu)>"
  Bus Selector1/1 -> Excitation System/3  "<Stator voltage  vq (pu)>"
  Machine 8 1000 MVA 22 kV/1 -> Bus Selector1/1
  HTG/1 -> Machine 8 1000 MVA 22 kV/1
  Excitation System/1 -> Machine 8 1000 MVA 22 kV/2
  wref/1 -> HTG/1
  Pref/1 -> HTG/2
  Vref/1 -> Excitation System/1
  HTG/2 -> Terminator5/1
  Ground/1 -> Excitation System/4
  connections:
  Machine 8 1000 MVA 22 kV/RConn3 -- Bus 37/LConn3
  Machine 8 1000 MVA 22 kV/RConn2 -- Bus 37/LConn2
  Machine 8 1000 MVA 22 kV/RConn1 -- Bus 37/LConn1
  5 MW/LConn3 -- Bus 37/RConn3 -- Transformer 8 772.2 MVA 22 kV / 345 kV/LConn3
  5 MW/LConn2 -- Bus 37/RConn2 -- Transformer 8 772.2 MVA 22 kV / 345 kV/LConn2
  5 MW/LConn1 -- Bus 37/RConn1 -- Load Flow Bus/LConn1 -- Transformer 8 772.2 MVA 22 kV / 345 kV/LConn1
  GT1_CB11/LConn1 -- Transformer 8 772.2 MVA 22 kV / 345 kV/RConn1
  GT1_CB11/LConn2 -- Transformer 8 772.2 MVA 22 kV / 345 kV/RConn2
  GT1_CB11/LConn3 -- Transformer 8 772.2 MVA 22 kV / 345 kV/RConn3
  C/RConn1 -- GT1_CB11/RConn3
  B/RConn1 -- GT1_CB11/RConn2
  A/RConn1 -- GT1_CB11/RConn1

== system IEEE39bus/SS_NorthSystem1/GT 9 ==
  5 MW : powerlib/Elements/Three-Phase Parallel RLC Load  LConnTagsString=A|B|C  Configuration=Y (grounded)  NominalVoltage=22e3  NominalFrequency=50  ActivePower=5e6  InductivePower=0  CapacitivePower=0  Measurements=None  LoadType=constant Z
  Bus Selector1 : BusSelector  OutputSignals="dq0 components.Stator voltage  vq (pu),dq0 components.Stator voltage  vd (pu),Mechanical.Rotor speed  wm  (pu),Mechanical.Rotor speed deviation  dw (pu),Output active power   Peo (pu),Output reactive power  Qeo (pu)"
  Bus 38 : powerlib/Measurements/Three-Phase V-I Measurement  VoltageMeasurement=phase-to-ground  SetLabelV=on  LabelV=V_bus_G9  Vpu=off  VpuLL=off  CurrentMeasurement=no  SetLabelI=on  LabelI=I_bus_G9  Ipu=off  Pbase=100e6  Vbase=16.5e3  OutputType=Complex  PhasorSimulation=off  PSBequivalent=0
  Excitation System : sps_avr/Excitation System  tr=20e-3  reg=[ 200, 0.02 ]  exc=[ 1, 0 .19]  tgr=[ 0, 0 ]  damp=[ 0.0012, 1 ]  sat=[ 0, 0 ]  lim=[ 0, 7.32, 0 ]  v0=[1.0156 1.6973]
  GT1_CB12 : Subsystem
  Ground : Ground
  HTG : powerlib/Machines/Hydraulic Turbine and Governor  sm="[ 10/3  0.07 ]"  gate="[  0.01  0.97518  -0.1  0.1 ]"  reg="[  0.05  1.163  0.105  0  0.01  ]"  hyd="[  0  2.67  ]"  dref=0  po=0.654
  Load Flow Bus : powerlib/Measurements/Load Flow Bus  LConnTagsString=a  ID=Bus-38  Vbase=22000  Vref=1.0265  Vangle=0  VLF=1.016  angleLF=1.986
      settings: AttributesFormatString=%<ID>\n%<Vbase>V\n%<VLF>pu\n%<angleLF>deg.
  Machine 9 1000 MVA 22 kV : powerlib/Machines/Synchronous Machine pu Standard  PresetModel=No  MechanicalLoad=Mechanical power Pm  ShowDetailedParameters=on  RotorType=Round  Units=per unit standard parameters  MeasurementBus=off  NominalParameters="[ 1000E6  22000   50 ]"  Reactances1=[ 1.7901 0.4845 0.242 1.742 0.4989 0.242 0.03 ]  Reactances2=[ 0.995, 0.195, 0.155, 0.568, 0.143, 0.16 ]  dAxisTimeConstants=Open-circuit  qAxisTimeConstants=Open-circuit  TimeConstants1=[]  TimeConstants2=[4.79 0.03 1.96 0.04]  TimeConstants3=[]  TimeConstants4=[]  TimeConstants5=[ 9.2, 0.01, 0.01 ]  TimeConstants6=[]  TimeConstants7=[]  TimeConstants8=[]  StatorResistance=0.005  Mechanical=[ 4.058 0.02 20]  PolePairs=20  InitialConditions=[0 -39.4462 0.720476 0.720476 0.720476 -1.93203 -121.932 118.068 1.69726]  SetSaturation=off  Saturation=[0.6404,0.7127,0.8441,0.9214,0.9956,1.082,1.19,1.316,1.457;0.7,0.7698,0.8872,0.9466,0.9969,1.046,1.1,1.151,1.201]  LoadFlowParameters=[1 830000000 22583 0]  TsPowergui=0  TsBlock=-1  IterativeModel=Trapezoidal non iterative  BusType=PV  Pref=7.3e+008  Qref=0  Qmin=-500e6  Qmax=50e6  PLF=0  QLF=0
      settings: AttributesFormatString=\n\n
  Terminator5 : Terminator
  Transformer 9 935 MVA 22 kV / 345 kV : powerlib/Elements/Three-Phase Transformer (Two Windings)  Winding1Connection=Delta (D1)  Winding2Connection=Yg  CoreType=Three single-phase transformers  SetSaturation=off  Hysteresis=off  DataFile='hysteresis'  SetInitialFlux=off  Measurements=None  UNITS=pu  NominalPower=[ 935e6 50 ]  Winding1="[ 22e3  0.0008*935/100/2  0.0156*935/100/2]"  Winding2="[ 1.025*345e3  0.0008*935/100/2  0.0156*935/100/2]"  Rm=500  Lm=500  L0=0.5  Saturation="[ 0,0  ;  0.005,1.2  ;  1.0,1.4 ]"  InitialFluxes=[ 0.8 , -0.8 , 0.7 ]  MoreParameters=off  BreakLoop=off  DataType=off  TransfoNumber=0
  wref : Constant
  wref1 : Constant  Value=0.654
  wref2 : Constant  Value=1.0265
  A : PMIOPort  Port=1  Side=Right
  B : PMIOPort  Port=2  Side=Right
  C : PMIOPort  Port=3  Side=Right
  tag scope: P_G9=global, Q_G9=global, V_G9=global, Wm_G9=global
  wires:
  Ground/1 -> Excitation System/4
  HTG/2 -> Terminator5/1
  wref2/1 -> Excitation System/1
  wref1/1 -> HTG/2
  wref/1 -> HTG/1
  Excitation System/1 -> Machine 9 1000 MVA 22 kV/2
  HTG/1 -> Machine 9 1000 MVA 22 kV/1
  Machine 9 1000 MVA 22 kV/1 -> Bus Selector1/1
  Bus Selector1/1 -> Excitation System/3  "<Stator voltage  vq (pu)>"
  Bus Selector1/2 -> Excitation System/2  "<Stator voltage  vd (pu)>"
  Bus Selector1/3 -> HTG/3, [Wm_G9]  "<Rotor speed  wm  (pu)>"
  Bus Selector1/4 -> HTG/5  "<Rotor speed deviation  dw (pu)>"
  Bus Selector1/5 -> HTG/4, [P_G9]  "<Output active power   Peo (pu)>"
  Bus Selector1/6 -> [Q_G9]  "<Output reactive power  Qeo (pu)>"
  [V_bus_G9] -> [V_G9]
  connections:
  Transformer 9 935 MVA 22 kV / 345 kV/LConn1 -- Load Flow Bus/LConn1 -- Bus 38/RConn1 -- 5 MW/LConn1
  Transformer 9 935 MVA 22 kV / 345 kV/LConn2 -- Bus 38/RConn2 -- 5 MW/LConn2
  Transformer 9 935 MVA 22 kV / 345 kV/LConn3 -- Bus 38/RConn3 -- 5 MW/LConn3
  Machine 9 1000 MVA 22 kV/RConn1 -- Bus 38/LConn1
  Machine 9 1000 MVA 22 kV/RConn2 -- Bus 38/LConn2
  Machine 9 1000 MVA 22 kV/RConn3 -- Bus 38/LConn3
  Transformer 9 935 MVA 22 kV / 345 kV/RConn2 -- GT1_CB12/LConn2
  Transformer 9 935 MVA 22 kV / 345 kV/RConn1 -- GT1_CB12/LConn1
  Transformer 9 935 MVA 22 kV / 345 kV/RConn3 -- GT1_CB12/LConn3
  B/RConn1 -- GT1_CB12/RConn2
  C/RConn1 -- GT1_CB12/RConn3
  A/RConn1 -- GT1_CB12/RConn1

== system IEEE39bus/SS_NorthSystem1/Load 25 ==
  Terminator : Terminator
  Three-Phase Dynamic Load : powerlib/Elements/Three-Phase Dynamic Load  NominalVoltage="[345e3  50 ]"  ActiveReactivePowers=[2.24e+08 4.72e+07]  PositiveSequence=[1.03404 25.0543]  ExternalControl=on  NpNq=[0 0]  TimeConstants="[0  0  0  0]"  MinimumVoltage=0.7  LoadFlowParameters=[4,0,0,0,0]
  V_Bus_L25 : powerlib/Measurements/Three-Phase V-I Measurement  VoltageMeasurement=phase-to-ground  SetLabelV=off  LabelV=V_Bus_L25  Vpu=off  VpuLL=off  CurrentMeasurement=yes  SetLabelI=on  LabelI=I_L25  Ipu=off  Pbase=100e6  Vbase=230e3  OutputType=Complex  PhasorSimulation=off  PSBequivalent=0
  A : PMIOPort  Port=1  Side=Left
  B : PMIOPort  Port=2  Side=Left
  C : PMIOPort  Port=3  Side=Left
  tag scope: V_L25=global
  wires:
  Three-Phase Dynamic Load/1 -> Terminator/1
  V_Bus_L25/1 -> [V_L25]
  [load25] -> Three-Phase Dynamic Load/1
  connections:
  V_Bus_L25/RConn1 -- Three-Phase Dynamic Load/LConn1
  C/RConn1 -- V_Bus_L25/LConn3
  B/RConn1 -- V_Bus_L25/LConn2
  A/RConn1 -- V_Bus_L25/LConn1
  V_Bus_L25/RConn2 -- Three-Phase Dynamic Load/LConn2
  V_Bus_L25/RConn3 -- Three-Phase Dynamic Load/LConn3

== system IEEE39bus/SS_NorthSystem1/Load 26 ==
  Bus_L26 : powerlib/Measurements/Three-Phase V-I Measurement  VoltageMeasurement=phase-to-ground  SetLabelV=off  LabelV=V_Bus_L26  Vpu=off  VpuLL=off  CurrentMeasurement=yes  SetLabelI=on  LabelI=I_L26  Ipu=off  Pbase=100e6  Vbase=230e3  OutputType=Complex  PhasorSimulation=off  PSBequivalent=0
  Terminator : Terminator
  Three-Phase Dynamic Load : powerlib/Elements/Three-Phase Dynamic Load  NominalVoltage=[345e3 50 ]  ActiveReactivePowers=[1.39e+08 1.7e+07]  PositiveSequence=[1.02673 21.7857]  ExternalControl=on  NpNq=[0 0]  TimeConstants="[0  0  0  0]"  MinimumVoltage=0.7  LoadFlowParameters=[4,0,0,0,0]
  A : PMIOPort  Port=1  Side=Left
  B : PMIOPort  Port=2  Side=Left
  C : PMIOPort  Port=3  Side=Left
  tag scope: V_L26=global
  wires:
  Three-Phase Dynamic Load/1 -> Terminator/1
  Bus_L26/1 -> [V_L26]
  [load26] -> Three-Phase Dynamic Load/1
  connections:
  Three-Phase Dynamic Load/LConn1 -- Bus_L26/RConn1
  C/RConn1 -- Bus_L26/LConn3
  B/RConn1 -- Bus_L26/LConn2
  A/RConn1 -- Bus_L26/LConn1
  Bus_L26/RConn2 -- Three-Phase Dynamic Load/LConn2
  Bus_L26/RConn3 -- Three-Phase Dynamic Load/LConn3

== system IEEE39bus/SS_NorthSystem1/Load 28 ==
  Bus_L28 : powerlib/Measurements/Three-Phase V-I Measurement  VoltageMeasurement=phase-to-ground  SetLabelV=off  LabelV=V_Bus_L28  Vpu=off  VpuLL=off  CurrentMeasurement=yes  SetLabelI=on  LabelI=I_L28  Ipu=off  Pbase=100e6  Vbase=230e3  OutputType=Complex  PhasorSimulation=off  PSBequivalent=0
  Terminator : Terminator
  Three-Phase Dynamic Load : powerlib/Elements/Three-Phase Dynamic Load  NominalVoltage=[345e3 50]  ActiveReactivePowers=[2.06e+08 2.76e+07]  PositiveSequence=[1.03092 23.6623]  ExternalControl=on  NpNq=[0 0]  TimeConstants="[0  0  0  0]"  MinimumVoltage=0.7  LoadFlowParameters=[4,0,0,0,0]
  A : PMIOPort  Port=1  Side=Left
  B : PMIOPort  Port=2  Side=Left
  C : PMIOPort  Port=3  Side=Left
  tag scope: V_L28=global
  wires:
  Three-Phase Dynamic Load/1 -> Terminator/1
  Bus_L28/1 -> [V_L28]
  [load28] -> Three-Phase Dynamic Load/1
  connections:
  Bus_L28/RConn3 -- Three-Phase Dynamic Load/LConn3
  Bus_L28/RConn2 -- Three-Phase Dynamic Load/LConn2
  A/RConn1 -- Bus_L28/LConn1
  B/RConn1 -- Bus_L28/LConn2
  C/RConn1 -- Bus_L28/LConn3
  Bus_L28/RConn1 -- Three-Phase Dynamic Load/LConn1

== system IEEE39bus/SS_NorthSystem1/Load 29 ==
  Bus_L29 : powerlib/Measurements/Three-Phase V-I Measurement  VoltageMeasurement=phase-to-ground  SetLabelV=off  LabelV=V_Bus_L29  Vpu=off  VpuLL=off  CurrentMeasurement=yes  SetLabelI=on  LabelI=I_L29  Ipu=off  Pbase=100e6  Vbase=230e3  OutputType=Complex  PhasorSimulation=off  PSBequivalent=0
  Terminator : Terminator
  Three-Phase Dynamic Load : powerlib/Elements/Three-Phase Dynamic Load  NominalVoltage=[345e3 50 ]  ActiveReactivePowers=[2.835e+08 2.69e+07]  PositiveSequence=[1.03368 25.6776]  ExternalControl=on  NpNq=[0 0]  TimeConstants="[0  0  0  0]"  MinimumVoltage=0.7  LoadFlowParameters=[4,0,0,0,0]
  A : PMIOPort  Port=1  Side=Left
  B : PMIOPort  Port=2  Side=Left
  C : PMIOPort  Port=3  Side=Left
  tag scope: V_L29=global
  wires:
  Three-Phase Dynamic Load/1 -> Terminator/1
  Bus_L29/1 -> [V_L29]
  [load29] -> Three-Phase Dynamic Load/1
  connections:
  Three-Phase Dynamic Load/LConn1 -- Bus_L29/RConn1
  C/RConn1 -- Bus_L29/LConn3
  B/RConn1 -- Bus_L29/LConn2
  A/RConn1 -- Bus_L29/LConn1
  Bus_L29/RConn2 -- Three-Phase Dynamic Load/LConn2
  Bus_L29/RConn3 -- Three-Phase Dynamic Load/LConn3

== system IEEE39bus/SS_NorthSystem1/Machines Measurements ==
  Mux : Mux  Inputs=2
  Mux1 : Mux
  Mux2 : Mux
  Machines Measurements : Outport
  wires:
  Mux2/1 -> Mux/2
  Mux1/1 -> Mux/1
  Mux/1 -> Machines Measurements/1
  [Wm_G9] -> Mux2/4
  [Q_G9] -> Mux2/3
  [P_G9] -> Mux2/2
  [V_G9] -> Mux2/1
  [Wm_G8] -> Mux1/4
  [Q_G8] -> Mux1/3
  [P_G8] -> Mux1/2
  [V_G8] -> Mux1/1

== system IEEE39bus/SS_NorthSystem2/Buses current_N ==
  Mux3 : Mux  Inputs=6
  curremt : Outport
  wires:
  [I_bus_1] -> Mux3/1
  [I_bus_2] -> Mux3/2
  [I_L3] -> Mux3/3
  [I_bus_17] -> Mux3/4
  [I_L18] -> Mux3/5
  Mux3/1 -> curremt/1
  [I_L27] -> Mux3/6

== system IEEE39bus/SS_NorthSystem2/Buses voltages_N ==
  Mux3 : Mux  Inputs=6
  Voltages : Outport
  wires:
  Mux3/1 -> Voltages/1
  [V_L27] -> Mux3/6
  [V_L18] -> Mux3/5
  [V_bus_17] -> Mux3/4
  [V_L3] -> Mux3/3
  [V_bus_2] -> Mux3/2
  [V_bus_1] -> Mux3/1

== system IEEE39bus/SS_NorthSystem2/GT 10 ==
  5 MW : powerlib/Elements/Three-Phase Parallel RLC Load  LConnTagsString=A|B|C  Configuration=Y (grounded)  NominalVoltage=22e3  NominalFrequency=50  ActivePower=5e6  InductivePower=0  CapacitivePower=0  Measurements=None  LoadType=constant Z
  Bus Selector1 : BusSelector  OutputSignals="dq0 components.Stator voltage  vq (pu),dq0 components.Stator voltage  vd (pu),Mechanical.Rotor speed  wm  (pu),Mechanical.Rotor speed deviation  dw (pu),Output active power   Peo (pu),Output reactive power  Qeo (pu)"
  Bus 30 : powerlib/Measurements/Three-Phase V-I Measurement  VoltageMeasurement=phase-to-ground  SetLabelV=on  LabelV=V_bus_G10  Vpu=off  VpuLL=off  CurrentMeasurement=no  SetLabelI=on  LabelI=I_bus_G10  Ipu=off  Pbase=100e6  Vbase=16.5e3  OutputType=Complex  PhasorSimulation=off  PSBequivalent=0
  Excitation System : sps_avr/Excitation System  tr=20e-3  reg=[ 200, 0.02 ]  exc=[ 1, 0 .19]  tgr=[ 0, 0 ]  damp=[ 0.0012, 1 ]  sat=[ 0, 0 ]  lim=[ 0, 7.32, 0 ]  v0=[1.025 1.2732]
  GT1_CB14 : Subsystem
  Ground : Ground
  HTG : powerlib/Machines/Hydraulic Turbine and Governor  sm="[ 10/3  0.07 ]"  gate="[  0.01  0.97518  -0.1  0.1 ]"  reg="[  0.05  1.163  0.105  0  0.01  ]"  hyd="[  0  2.67  ]"  dref=0  po=0.324
  Load Flow Bus : powerlib/Measurements/Load Flow Bus  LConnTagsString=a  ID=Bus-30  Vbase=22000  Vref=1.025  Vangle=0  VLF=1.025  angleLF=-2.488
      settings: AttributesFormatString=%<ID>\n%<Vbase>V\n%<VLF>pu\n%<angleLF>deg.
  Machine 10 1000 MVA 22 kV : powerlib/Machines/Synchronous Machine pu Standard  PresetModel=No  MechanicalLoad=Mechanical power Pm  ShowDetailedParameters=on  RotorType=Round  Units=per unit standard parameters  MeasurementBus=off  NominalParameters="[ 1000E6  22000   50 ]"  Reactances1="[ 1.29 0.4 0.2 0.89 0.103 0.2 0.013  ]"  Reactances2=[ 0.995, 0.195, 0.155, 0.568, 0.143, 0.16 ]  dAxisTimeConstants=Open-circuit  qAxisTimeConstants=Open-circuit  TimeConstants1=[]  TimeConstants2=[10.2 0.03 0.02 0.04]  TimeConstants3=[]  TimeConstants4=[]  TimeConstants5=[ 9.2, 0.01, 0.01 ]  TimeConstants6=[]  TimeConstants7=[]  TimeConstants8=[]  StatorResistance=0.005  Mechanical=[ 3.255 0.02 20]  PolePairs=20  InitialConditions=[0 -77.6756 0.367118 0.367118 0.367118 -24.0341 -144.034 95.9659 1.27317]  SetSaturation=off  Saturation=[0.6404,0.7127,0.8441,0.9214,0.9956,1.082,1.19,1.316,1.457;0.7,0.7698,0.8872,0.9466,0.9969,1.046,1.1,1.151,1.201]  LoadFlowParameters=[1 632000000 21938.4 0]  TsPowergui=0  TsBlock=-1  IterativeModel=Trapezoidal non iterative  BusType=PV  Pref=3.5e+008  Qref=0  Qmin=-500e6  Qmax=200e6  PLF=0  QLF=0
      settings: AttributesFormatString=\n\n
  Pref : Constant  Value=0.324
  Terminator5 : Terminator
  Transformer 10  1419 MVA 22 kV / 345 kV : powerlib/Elements/Three-Phase Transformer (Two Windings)  Winding1Connection=Delta (D1)  Winding2Connection=Yg  CoreType=Three single-phase transformers  SetSaturation=off  Hysteresis=off  DataFile='hysteresis'  SetInitialFlux=off  Measurements=None  UNITS=pu  NominalPower=[ 1419e6 50 ]  Winding1="[ 22e3   0    0.0181*1419/100/2 ]"  Winding2=|  Rm=500  Lm=500  L0=0.5  Saturation="[ 0,0  ;  0.005,1.2  ;  1.0,1.4 ]"  InitialFluxes=[ 0.8 , -0.8 , 0.7 ]  MoreParameters=off  BreakLoop=off  DataType=off  TransfoNumber=0
      | [ 1.025*345e3 0    0.0181*1419/100/2
      | ]
  Vref : Constant  Value=1.025
  wref : Constant
  A : PMIOPort  Port=1  Side=Right
  B : PMIOPort  Port=2  Side=Right
  C : PMIOPort  Port=3  Side=Right
  tag scope: P_G10=global, Q_G10=global, V_G10=global, Wm_G10=global
  wires:
  Ground/1 -> Excitation System/4
  HTG/2 -> Terminator5/1
  Vref/1 -> Excitation System/1
  Pref/1 -> HTG/2
  wref/1 -> HTG/1
  Excitation System/1 -> Machine 10 1000 MVA 22 kV/2
  HTG/1 -> Machine 10 1000 MVA 22 kV/1
  Machine 10 1000 MVA 22 kV/1 -> Bus Selector1/1
  Bus Selector1/1 -> Excitation System/3  "<Stator voltage  vq (pu)>"
  Bus Selector1/2 -> Excitation System/2  "<Stator voltage  vd (pu)>"
  Bus Selector1/3 -> HTG/3, [Wm_G10]  "<Rotor speed  wm  (pu)>"
  Bus Selector1/4 -> HTG/5  "<Rotor speed deviation  dw (pu)>"
  Bus Selector1/5 -> HTG/4, [P_G10]  "<Output active power   Peo (pu)>"
  Bus Selector1/6 -> [Q_G10]  "<Output reactive power  Qeo (pu)>"
  [V_bus_G10] -> [V_G10]
  connections:
  Transformer 10  1419 MVA 22 kV / 345 kV/LConn1 -- Load Flow Bus/LConn1 -- Bus 30/RConn1 -- 5 MW/LConn1
  Transformer 10  1419 MVA 22 kV / 345 kV/LConn2 -- Bus 30/RConn2 -- 5 MW/LConn2
  Transformer 10  1419 MVA 22 kV / 345 kV/LConn3 -- Bus 30/RConn3 -- 5 MW/LConn3
  Machine 10 1000 MVA 22 kV/RConn1 -- Bus 30/LConn1
  Machine 10 1000 MVA 22 kV/RConn2 -- Bus 30/LConn2
  Machine 10 1000 MVA 22 kV/RConn3 -- Bus 30/LConn3
  GT1_CB14/LConn1 -- Transformer 10  1419 MVA 22 kV / 345 kV/RConn1
  GT1_CB14/LConn2 -- Transformer 10  1419 MVA 22 kV / 345 kV/RConn2
  GT1_CB14/LConn3 -- Transformer 10  1419 MVA 22 kV / 345 kV/RConn3
  A/RConn1 -- GT1_CB14/RConn1
  C/RConn1 -- GT1_CB14/RConn3
  B/RConn1 -- GT1_CB14/RConn2

== system IEEE39bus/SS_NorthSystem2/Load 18 ==
  Bus_L18 : powerlib/Measurements/Three-Phase V-I Measurement  VoltageMeasurement=phase-to-ground  SetLabelV=off  LabelV=V_Bus_L18  Vpu=off  VpuLL=off  CurrentMeasurement=yes  SetLabelI=on  LabelI=I_L18  Ipu=off  Pbase=100e6  Vbase=230e3  OutputType=Complex  PhasorSimulation=off  PSBequivalent=0
  Terminator : Terminator
  Three-Phase Dynamic Load : powerlib/Elements/Three-Phase Dynamic Load  NominalVoltage=[345e3 50 ]  ActiveReactivePowers=[1.58e+08 3e+07]  PositiveSequence=[1.0086 19.7218]  ExternalControl=on  NpNq=[0 0]  TimeConstants="[0  0  0  0]"  MinimumVoltage=0.7  LoadFlowParameters=[4,0,0,0,0]
  A : PMIOPort  Port=1  Side=Left
  B : PMIOPort  Port=2  Side=Left
  C : PMIOPort  Port=3  Side=Left
  tag scope: V_L18=global
  wires:
  Three-Phase Dynamic Load/1 -> Terminator/1
  Bus_L18/1 -> [V_L18]
  [load18] -> Three-Phase Dynamic Load/1
  connections:
  Bus_L18/RConn3 -- Three-Phase Dynamic Load/LConn3
  Bus_L18/RConn2 -- Three-Phase Dynamic Load/LConn2
  A/RConn1 -- Bus_L18/LConn1
  B/RConn1 -- Bus_L18/LConn2
  C/RConn1 -- Bus_L18/LConn3
  Bus_L18/RConn1 -- Three-Phase Dynamic Load/LConn1

== system IEEE39bus/SS_NorthSystem2/Load 27 ==
  Bus_L27 : powerlib/Measurements/Three-Phase V-I Measurement  VoltageMeasurement=phase-to-ground  SetLabelV=off  LabelV=V_Bus_L27  Vpu=off  VpuLL=off  CurrentMeasurement=yes  SetLabelI=on  LabelI=I_L27  Ipu=off  Pbase=100e6  Vbase=230e3  OutputType=Complex  PhasorSimulation=off  PSBequivalent=0
  Terminator : Terminator
  Three-Phase Dynamic Load : powerlib/Elements/Three-Phase Dynamic Load  NominalVoltage=[345e3 50]  ActiveReactivePowers=[2.81e+08 7.55e+07]  PositiveSequence=[1.0131 19.7618]  ExternalControl=on  NpNq=[0 0]  TimeConstants="[0  0  0  0]"  MinimumVoltage=0.7  LoadFlowParameters=[4,0,0,0,0]
  A : PMIOPort  Port=1  Side=Left
  B : PMIOPort  Port=2  Side=Left
  C : PMIOPort  Port=3  Side=Left
  tag scope: V_L27=global
  wires:
  Three-Phase Dynamic Load/1 -> Terminator/1
  Bus_L27/1 -> [V_L27]
  [load27] -> Three-Phase Dynamic Load/1
  connections:
  Bus_L27/RConn3 -- Three-Phase Dynamic Load/LConn3
  Bus_L27/RConn2 -- Three-Phase Dynamic Load/LConn2
  A/RConn1 -- Bus_L27/LConn1
  B/RConn1 -- Bus_L27/LConn2
  C/RConn1 -- Bus_L27/LConn3
  Three-Phase Dynamic Load/LConn1 -- Bus_L27/RConn1

== system IEEE39bus/SS_NorthSystem2/Load 3 ==
  Bus_L3 : powerlib/Measurements/Three-Phase V-I Measurement  VoltageMeasurement=phase-to-ground  SetLabelV=off  LabelV=V_Bus_L3  Vpu=off  VpuLL=off  CurrentMeasurement=yes  SetLabelI=on  LabelI=I_L3  Ipu=off  Pbase=100e6  Vbase=230e3  OutputType=Complex  PhasorSimulation=off  PSBequivalent=0
  Terminator : Terminator
  Three-Phase Dynamic Load : powerlib/Elements/Three-Phase Dynamic Load  NominalVoltage=[ 345e3 50 ]  ActiveReactivePowers=[5e+07 2.5e+07]  PositiveSequence=[1.01048 21.0012]  ExternalControl=on  NpNq=[0 0]  TimeConstants="[0  0  0  0]"  MinimumVoltage=0.7  LoadFlowParameters=[4,0,0,0,0]
  A : PMIOPort  Port=1  Side=Left
  B : PMIOPort  Port=2  Side=Left
  C : PMIOPort  Port=3  Side=Left
  tag scope: V_L3=global
  wires:
  Three-Phase Dynamic Load/1 -> Terminator/1
  Bus_L3/1 -> [V_L3]
  [load3] -> Three-Phase Dynamic Load/1
  connections:
  Bus_L3/RConn1 -- Three-Phase Dynamic Load/LConn1
  C/RConn1 -- Bus_L3/LConn3
  B/RConn1 -- Bus_L3/LConn2
  A/RConn1 -- Bus_L3/LConn1
  Bus_L3/RConn2 -- Three-Phase Dynamic Load/LConn2
  Bus_L3/RConn3 -- Three-Phase Dynamic Load/LConn3

== system IEEE39bus/SS_NorthSystem2/Machines Measurements ==
  Mux : Mux  Inputs=1
  Mux3 : Mux
  Machines Measurements : Outport
  wires:
  Mux3/1 -> Mux/1
  [Wm_G10] -> Mux3/4
  [Q_G10] -> Mux3/3
  [P_G10] -> Mux3/2
  [V_G10] -> Mux3/1
  Mux/1 -> Machines Measurements/1

== system IEEE39bus/SS_WestSystem1/Buses Current_W ==
  Mux3 : Mux  Inputs=5
  Current : Outport
  wires:
  Mux3/1 -> Current/1
  [I_L4] -> Mux3/1
  [I_bus_5] -> Mux3/2
  [I_L8] -> Mux3/3
  [I_bus_9] -> Mux3/4
  [I_L39] -> Mux3/5

== system IEEE39bus/SS_WestSystem1/Buses voltages_W ==
  Mux3 : Mux  Inputs=5
  Voltages : Outport
  wires:
  [V_L39] -> Mux3/5
  [V_bus_9] -> Mux3/4
  [V_L8] -> Mux3/3
  [V_bus_5] -> Mux3/2
  [V_L4] -> Mux3/1
  Mux3/1 -> Voltages/1
